simulink model "trigger_test"  (R2017a)
settings: Solver=FixedStepAuto  StartTime=0.0  StopTime=inf  RelTol=1e-3  EnableMultiTasking=on
undefined symbols (not defined in the file): Green, led0, sigbuilder_block
libraries: embdlinuxlib x2
settings Model: Creator=Vincent  LastModifiedBy=Vincent
settings SolverCC: PositivePriorityOrder=on
settings OptimizationCC: PassReuseOutputArgsAs=Individual arguments  MaxStackSize=64
settings DebuggingCC: ParameterTunabilityLossMsg=error
settings HardwareCC: ProdBitPerPointer=32  ProdBitPerSizeT=32  ProdBitPerPtrDiffT=32  ProdLargestAtomicInteger=Long  ProdLargestAtomicFloat=Double  ProdWordSize=32  ProdHWDeviceType=ARM Compatible->ARM Cortex  UseEmbeddedCoderFeatures=off
settings SFSimCC: MATLABDynamicMemAlloc=off
settings RTWCC: SystemTargetFile=ert.tlc  HardwareBoard=Raspberry Pi  TLCOptions="-aInlineSetEventsForThisBaseRateFcn=TLC_FALSE -aSuppressMultiTaskScheduler=TLC_FALSE  -aRateBasedStepFcn=0"  TemplateMakefile=ert_default_tmf  Description=Embedded Coder  GenerateReport=on  Toolchain=GNU GCC Raspberry Pi  IncludeHyperlinkInReport=on  LaunchReport=on  GenerateTraceInfo=on  GenerateTraceReport=on  GenerateTraceReportSl=on  GenerateTraceReportSf=on  GenerateTraceReportEml=on
settings CodeAppCC: ForceParamTrailComments=on  IgnoreCustomStorageClasses=off  OperatorAnnotations=on  SimulinkDataObjDesc=on  SFDataObjDesc=on  MATLABFcnDesc=on  InsertBlockDesc=on  MATLABSourceComments=on
settings ERTTargetCC: SupportNonInlinedSFcns=on  SupportVariableSizeSignals=on

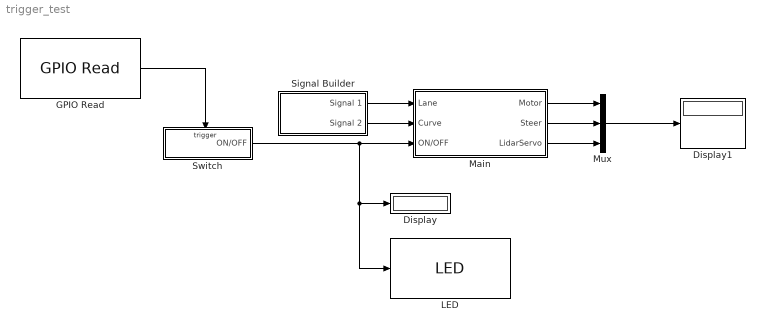
== system trigger_test ==
  Display : Display
  Display1 : Display
  GPIO Read : embdlinuxlib/GPIO Read  board=Model B+  gpio=22  internalResistor=Off  sampleTime=0.1  direction=Input  blockPlatform=Raspberry Pi
  LED : embdlinuxlib/LED  board=Model B+  led=led0 (Green)  blockPlatform=Raspberry Pi
  Main : Subsystem  TreatAsAtomicUnit=on
  Mux : Mux  Inputs=3
  Signal Builder : Subsystem  Tag=STV Subsys  LoadFcn=sigbuilder_block('load');  StartFcn=sigbuilder_block('start');  StopFcn=sigbuilder_block('stop');  ClipboardFcn=sigbuilder_block('clipboard');  mask(Sigbuilder block){tuvar=[0:10]}
      mask help: Simulink:masks:SigbuilderBlock_MD
      mask init:
      | if ~strcmp(get_param(bdroot(gcbh),'SimulationStatus'),'stopped') tuvar = sigbuilder_block('maskInit'); end
      settings: CopyFcn=sigbuilder_block('copy');  DeleteFcn=sigbuilder_block('delete');  ModelCloseFcn=sigbuilder_block('modelClose');  PreSaveFcn=sigbuilder_block('preSave');  PauseFcn=sigbuilder_block('pause');  ContinueFcn=sigbuilder_block('continue');  NameChangeFcn=sigbuilder_block('namechange');  OpenFcn=sigbuilder_block('open',[437.6 199.2 550.4 400 ]);  CloseFcn=sigbuilder_block('close');
      mask Display: plot(0, 0, 100, 100,[2, 2, 32, 32, 2], [68, 8, 8, 68, 68],[32, 2], [38, 38], [32, 19, 2],[53, 60, 44], [32, 17, 17, 2],[16, 16, 31, 31]);txt = getActiveGroup(gcbh);text(2, 100, txt,'verticalAlignment', 'top');
  Switch : Subsystem  TreatAsAtomicUnit=on
  wires:
  GPIO Read/1 -> Switch/Trigger
  Switch/1(ON/OFF) -> Display/1, LED/1, Main/3(ON/OFF)
  Main/1(Motor) -> Mux/1
  Main/2(Steer) -> Mux/2
  Main/3(LidarServo) -> Mux/3
  Mux/1 -> Display1/1
  Signal Builder/1(Signal 1) -> Main/1(Lane)
  Signal Builder/2(Signal 2) -> Main/2(Curve)

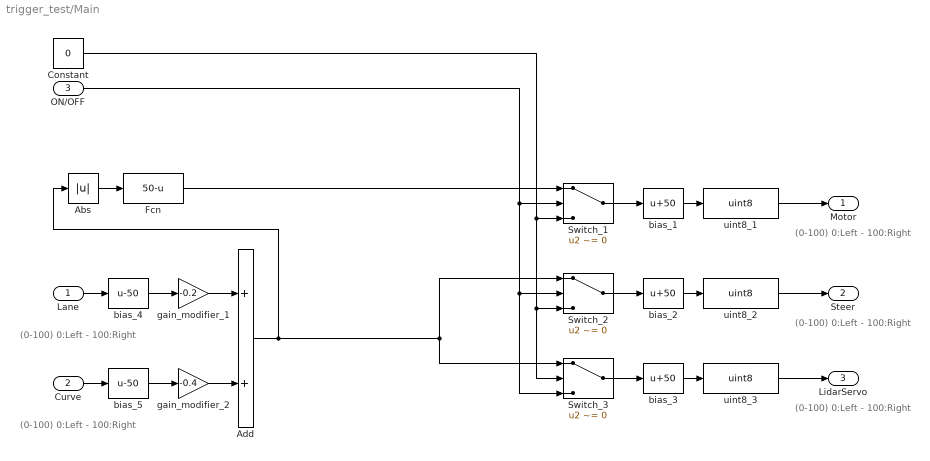
== system trigger_test/Main ==
  note: (0-100)
      | 0:Left - 100:Right
  note: (0-100)
      | 0:Left - 100:Right
  note: (0-100)
      | 0:Left - 100:Right
  note: (0-100)
      | 0:Left - 100:Right
  note: (0-100)
      | 0:Left - 100:Right
  Lane : Inport
  Curve : Inport  Port=2
  ON/OFF : Inport  Port=3
  Abs : Abs
  Add : Sum
  Constant : Constant  Value=0
  Fcn : Fcn  Expr=50-u
  Switch_1 : Switch  Criteria=u2 ~= 0
  Switch_2 : Switch  Criteria=u2 ~= 0
  Switch_3 : Switch  Criteria=u2 ~= 0
  bias_1 : Bias  Bias=50
  bias_2 : Bias  Bias=50
  bias_3 : Bias  Bias=50
  bias_4 : Bias  Bias=-50
  bias_5 : Bias  Bias=-50
  gain_modifier_1 : Gain  Gain=-0.2
  gain_modifier_2 : Gain  Gain=-0.4
  uint8_1 : DataTypeConversion  OutDataTypeStr=uint8
  uint8_2 : DataTypeConversion  OutDataTypeStr=uint8
  uint8_3 : DataTypeConversion  OutDataTypeStr=uint8
  Motor : Outport
  Steer : Outport  Port=2
  LidarServo : Outport  Port=3
  wires:
  uint8_2/1 -> Steer/1
  uint8_3/1 -> LidarServo/1
  bias_1/1 -> uint8_1/1
  uint8_1/1 -> Motor/1
  bias_2/1 -> uint8_2/1
  bias_3/1 -> uint8_3/1
  Lane/1 -> bias_4/1
  Curve/1 -> bias_5/1
  ON/OFF/1 -> Switch_3/3, Switch_2/2, Switch_1/2
  Constant/1 -> Switch_3/2, Switch_2/3, Switch_1/3
  Switch_3/1 -> bias_3/1
  Switch_2/1 -> bias_2/1
  Switch_1/1 -> bias_1/1
  bias_4/1 -> gain_modifier_1/1
  bias_5/1 -> gain_modifier_2/1
  gain_modifier_1/1 -> Add/1
  gain_modifier_2/1 -> Add/2
  Add/1 -> Abs/1, Switch_3/1, Switch_2/1
  Abs/1 -> Fcn/1
  Fcn/1 -> Switch_1/1

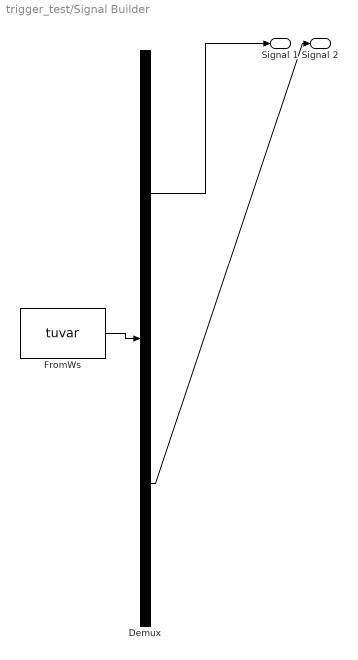
== system trigger_test/Signal Builder ==
  Demux : Demux  Tag=STV Demux  Outputs=2
  FromWs : FromWorkspace  Tag=STV FromWs  VariableName=tuvar  SampleTime=0
      SigBuilderData=|
      | common.afterFinalStr = 'Extrapolate'
      | common.sampleTime = 0
      | dataSet.timeRange = [0 10]
      | dataSet.name = 'Group 1'
      | sbobj.Groups.Name = 'Group 1'
      | sbobj.Groups.Signals(1).Name = 'Signal 1'
      | sbobj.Groups.Signals(1).XData = [0 1 2 3 4 10]
      | sbobj.Groups.Signals(1).YData = [0 0 50 -50 0 0]
      | sbobj.Groups.Signals(2).Name = 'Signal 2'
      | sbobj.Groups.Signals(2).XData = [0 6 7 8 9 10]
      | sbobj.Groups.Signals(2).YData = [0 0 50 -50 0 0]
  Signal 1 : Outport  Tag=STV Outport
  Signal 2 : Outport  Tag=STV Outport  Port=2
  wires:
  Demux/1 -> Signal 1/1
  FromWs/1 -> Demux/1
  Demux/2 -> Signal 2/1

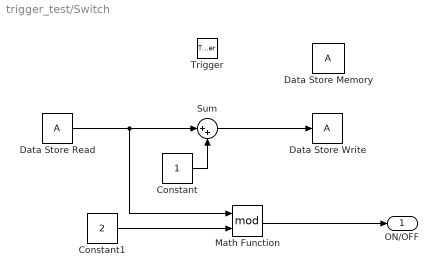
== system trigger_test/Switch ==
  Trigger : TriggerPort  VariantControl=Variant
  Constant : Constant
  Constant1 : Constant  Value=2
  Data Store Memory : DataStoreMemory  ReadBeforeWriteMsg=warning  WriteAfterWriteMsg=warning  WriteAfterReadMsg=warning  ShowAdditionalParam=off
  Data Store Read : DataStoreRead
  Data Store Write : DataStoreWrite
  Math Function : Math  Operator=mod  SaturateOnIntegerOverflow=on
  Sum : Sum  Inputs=|++
  ON/OFF : Outport
  wires:
  Sum/1 -> Data Store Write/1
  Data Store Read/1 -> Math Function/1, Sum/1
  Constant/1 -> Sum/2
  Constant1/1 -> Math Function/2
  Math Function/1 -> ON/OFF/1
